simulink model "state_space_w_kalman_3_ideal"  (R2018b)
settings: Solver=VariableStepAuto  StartTime=0.0  StopTime=simtime  RelTol=1e-3
undefined symbols (not defined in the file): g, kd_phi, ki_chi, kp_chi, kp_phi, vg
libraries: simulink_extras x2, simulink x1
settings Model: Creator=dino  LastModifiedBy=dino
settings SolverCC: ZeroCrossAlgorithm=Adaptive
settings DebuggingCC: IgnoredZcDiagnostic=none

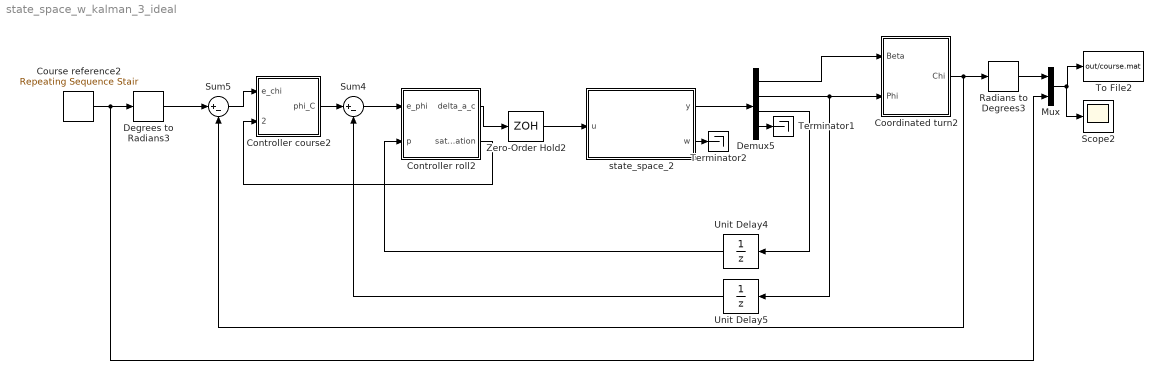
== system state_space_w_kalman_3_ideal ==
  Controller course2 : Subsystem
  Controller roll2 : Subsystem
  Coordinated turn2 : Subsystem
  Course reference2 : simulink/Sources/Repeating Sequence Stair  OutValues=step_series.'  tsamp=60  OutMin=[]  OutMax=[]  OutDataTypeStr=double  OutputDataTypeScalingMode=double  OutDataType=fixdt(0,8)  ConRadixGroup=Best Precision: Vector-wise  OutScaling=2^-12
  Degrees to Radians3 : simulink_extras/Transformations/Degrees to Radians
  Demux5 : Demux
  Mux : Mux  Inputs=2
  Radians to Degrees3 : simulink_extras/Transformations/Radians to Degrees
  Scope2 : Scope
  Sum4 : Sum  Inputs=|+-
  Sum5 : Sum  Inputs=|+-
  Terminator1 : Terminator
  Terminator2 : Terminator
  To File2 : ToFile  Filename=out/course.mat
  Unit Delay4 : UnitDelay  SampleTime=0.01
  Unit Delay5 : UnitDelay  SampleTime=0.01
  Zero-Order Hold2 : ZeroOrderHold  SampleTime=0.01
  state_space_2 : MATLAB Function  TreatAsAtomicUnit=on
  wires:
  Radians to Degrees3/1 -> Mux/1
  Demux5/3 -> Unit Delay4/1
  Demux5/4 -> Terminator1/1
  Zero-Order Hold2/1 -> state_space_2/1(u)
  Controller roll2/1(delta_a_c) -> Zero-Order Hold2/1
  Unit Delay4/1 -> Controller roll2/2(p)
  Coordinated turn2/1(Chi) -> Sum5/2, Radians to Degrees3/1
  Sum4/1 -> Controller roll2/1(e_phi)
  Unit Delay5/1 -> Sum4/2
  Course reference2/1 -> Degrees to Radians3/1, Mux/2
  Controller course2/1(phi_C) -> Sum4/1
  Sum5/1 -> Controller course2/1(e_chi)
  Degrees to Radians3/1 -> Sum5/1
  state_space_2/2(w) -> Terminator2/1
  Mux/1 -> Scope2/1, To File2/1
  state_space_2/1(y) -> Demux5/1
  Demux5/2 -> Unit Delay5/1, Coordinated turn2/2(Phi)
  Controller roll2/2(saturation) -> Controller course2/2(saturation)
  Demux5/1 -> Coordinated turn2/1(Beta)

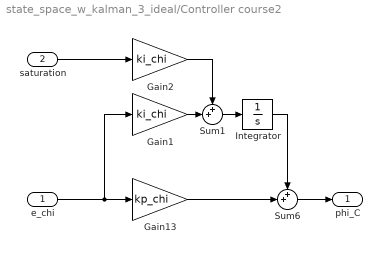
== system state_space_w_kalman_3_ideal/Controller course2 ==
  e_chi : Inport
  saturation : Inport  Port=2
  Gain1 : Gain  Gain=ki_chi
  Gain13 : Gain  Gain=kp_chi
  Gain2 : Gain  Gain=ki_chi
  Integrator : Integrator
  Sum1 : Sum  Inputs=++|
  Sum6 : Sum  Inputs=++|
  phi_C : Outport
  wires:
  Gain13/1 -> Sum6/2
  Sum6/1 -> phi_C/1
  e_chi/1 -> Gain1/1, Gain13/1
  Integrator/1 -> Sum6/1
  saturation/1 -> Gain2/1
  Gain1/1 -> Sum1/2
  Sum1/1 -> Integrator/1
  Gain2/1 -> Sum1/1

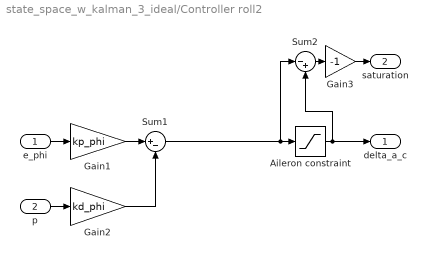
== system state_space_w_kalman_3_ideal/Controller roll2 ==
  e_phi : Inport
  p : Inport  Port=2
  "Aileron constraint " : Saturate  UpperLimit=30*deg2rad  LowerLimit=-30*deg2rad
  Gain1 : Gain  Gain=kp_phi
  Gain2 : Gain  Gain=kd_phi
  Gain3 : Gain  Gain=-1
  Sum1 : Sum  Inputs=|+-
  Sum2 : Sum  Inputs=|-+
  delta_a_c : Outport
  saturation : Outport  Port=2
  wires:
  Sum1/1 -> Sum2/1, "Aileron constraint "/1
  p/1 -> Gain2/1
  e_phi/1 -> Gain1/1
  "Aileron constraint "/1 -> delta_a_c/1, Sum2/2
  Gain1/1 -> Sum1/1
  Gain2/1 -> Sum1/2
  Sum2/1 -> Gain3/1
  Gain3/1 -> saturation/1

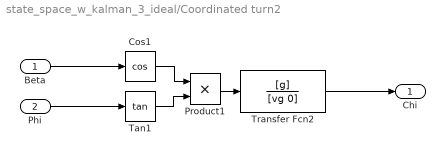
== system state_space_w_kalman_3_ideal/Coordinated turn2 ==
  Beta : Inport
  Phi : Inport  Port=2
  Cos1 : Trigonometry  Operator=cos
  Product1 : Product
  Tan1 : Trigonometry  Operator=tan
  Transfer Fcn2 : TransferFcn  Numerator=[g]  Denominator=[vg 0]
  Chi : Outport
  wires:
  Beta/1 -> Cos1/1
  Tan1/1 -> Product1/2
  Cos1/1 -> Product1/1
  Product1/1 -> Transfer Fcn2/1
  Phi/1 -> Tan1/1
  Transfer Fcn2/1 -> Chi/1

== matlab function state_space_w_kalman_3_ideal/state_space_2 ==
  data: u input; y output; w output
function [y, w] = state_space_3(u)
% Generate the output of the state space

    % Persistent variables to be kept between function calls
    persistent counter; % Variable for checking if it is the first iteration.
    persistent x;       % The state x
    
   % The next line is necessary for generating unique process noise for every simulation.
   % Otherwise, the noise will be equal every time you run the simulation,
   % even though it is white. This has to do with how Matlab generates
   % random numbers. 
   coder.extrinsic('randn','rng');
    
    h = 0.01;       % Time step of Euler integration
    delta_a_c = u;  % Aileron input
    
    if isempty(counter)
      % First iteration
        counter = 1;
           
        % Initialize state space
        x = zeros(5,1);
        w = zeros(5,1); 
        rng('shuffle'); % Necessary for generating unique process noise for every simulation.
    
    else
        % State-space matrices
        A = [-0.322, 0.052, 0.028, -1.12, 0.002;
             0, 0, 1, -0.001, 0;
             -10.6, 0, -2.87, 0.46, -0.65;  
             6.87, 0, -0.04, -0.32, -0.02;
             0, 0, 0, 0, -7.5];
 
        B = [0; 0; 0; 0; 7.5;];
        
        E = eye(5);
        
        % Discrete version
        Ad = eye(5) + h*A;
        Bd = h*B;
        Ed = E;
        
        % The Qd matrix in the assignment is given directly in discrete-time here and
        % therefore, it is not necessary to discretize E.
        Qd = h*10^-6*[0.001, 0, 0, 0, 0;
                  0, 1, 0, 0, 0;
                  0, 0, 100, 0, 0;
                  0, 0, 0, 10, 0;
                  0, 0, 0, 0, 0];
          
        w = 0*sqrt(Qd)*randn(5,1,1); % The standard deviation must be multiplied with random numbers with a zero-mean unit variance random number to generate process noise. 
        
        % Discrete-time state space update
        x = Ad*x + Bd * delta_a_c + Ed*w;
    end
    y = x(1:4); % Return every state except the actuator state.
end
